simulink model "P4E1OAAA"  (R2018a)
settings: Solver=FixedStepAuto  StartTime=0.0  StopTime=60  FixedStep=2.5  RelTol=1e-3  EnableMultiTasking=on
settings Model: Creator=CltControl  LastModifiedBy=Oscar
settings OptimizationCC: LifeSpan=inf
settings DebuggingCC: SFUnexpectedBacktrackingDiag=warning  SFNoUnconditionalDefaultTransitionDiag=warning  SFExecutionAtInitializationDiag=none
settings CodeAppCC: StateflowObjectComments=on
settings GRTTargetCC: TargetLangStandard=C89/C90 (ANSI)  GeneratePreprocessorConditionals=Disable all
settings ConfigComp: CovMetricSettings=dw  CovHtmlReporting=on  CovSaveCumulativeToWorkspaceVar=on  CovSaveSingleToWorkspaceVar=on  CovExternalEMLEnable=off

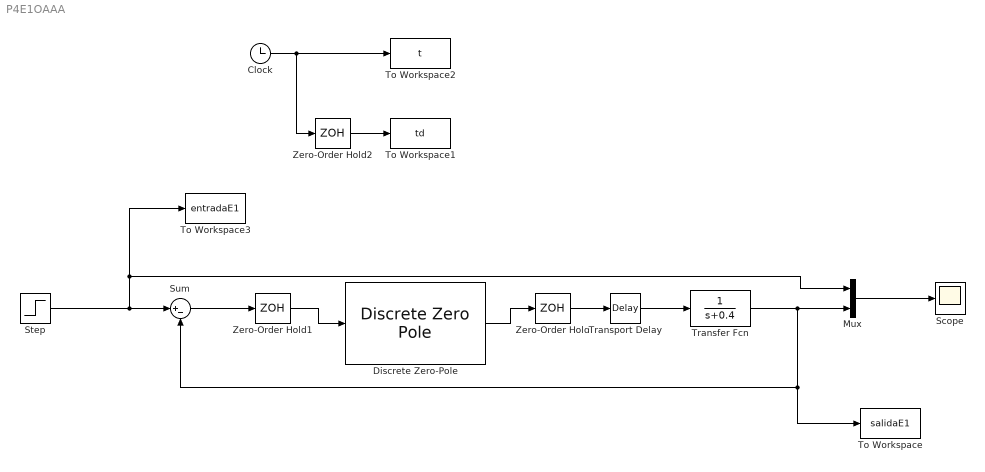
== system P4E1OAAA ==
  Clock : Clock
  Discrete Zero-Pole : DiscreteZeroPole  Zeros=[0.585]  Poles=[1]  Gain=0.21706  SampleTime=2.5
  Mux : Mux  Inputs=2
  Scope : Scope
  Step : Step  Time=0  SampleTime=2.5
  Sum : Sum  Inputs=|+-
  To Workspace : ToWorkspace  VariableName=salidaE1  SampleTime=-1
  To Workspace1 : ToWorkspace  VariableName=td  SampleTime=-1
  To Workspace2 : ToWorkspace  VariableName=t  SampleTime=-1
  To Workspace3 : ToWorkspace  VariableName=entradaE1  SampleTime=-1
  Transfer Fcn : TransferFcn  Denominator=[1 0.4]
  Transport Delay : TransportDelay  DelayTime=5
  Zero-Order Hold : ZeroOrderHold  SampleTime=2.5
  Zero-Order Hold1 : ZeroOrderHold  SampleTime=2.5
  Zero-Order Hold2 : ZeroOrderHold  SampleTime=2.5
  wires:
  Zero-Order Hold1/1 -> Discrete Zero-Pole/1
  Sum/1 -> Zero-Order Hold1/1
  Discrete Zero-Pole/1 -> Zero-Order Hold/1
  Clock/1 -> Zero-Order Hold2/1, To Workspace2/1
  Zero-Order Hold2/1 -> To Workspace1/1
  Zero-Order Hold/1 -> Transport Delay/1
  Transport Delay/1 -> Transfer Fcn/1
  Step/1 -> To Workspace3/1, Mux/1, Sum/1
  Mux/1 -> Scope/1
  Transfer Fcn/1 -> Sum/2, To Workspace/1, Mux/2
